simulink library "aoc"  (Simulink 8.1)
settings: Solver=ode45  StartTime=0.0  StopTime=10.0  RelTol=1e-3
settings Model: Creator=xsellart  LastModifiedBy=AT015555

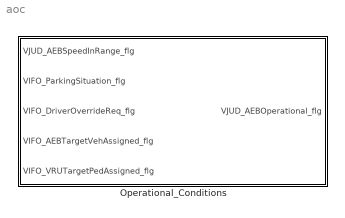
== system aoc ==
  Operational_Conditions : Subsystem

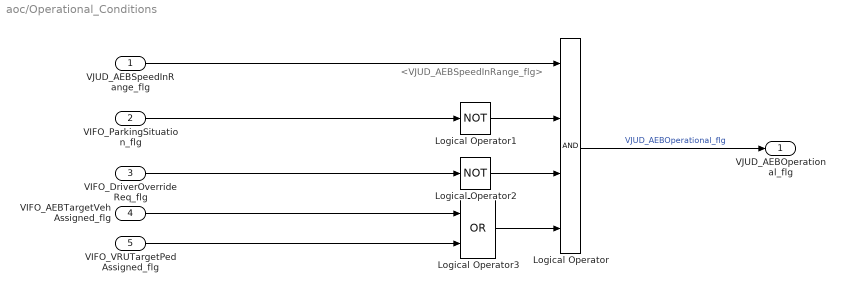
== system aoc/Operational_Conditions ==
  note: <VJUD_AEBSpeedInRange_flg>
  VJUD_AEBSpeedInRange_flg : Inport
  VIFO_ParkingSituation_flg : Inport  Port=2
  VIFO_DriverOverrideReq_flg : Inport  Port=3
  VIFO_AEBTargetVehAssigned_flg : Inport  Port=4
  VIFO_VRUTargetPedAssigned_flg : Inport  Port=5
  Logical Operator : Logic  Inputs=4  AllPortsSameDT=off  OutDataTypeStr=boolean
  Logical Operator1 : Logic  Operator=NOT  AllPortsSameDT=off  OutDataTypeStr=boolean
  Logical Operator2 : Logic  Operator=NOT  AllPortsSameDT=off  OutDataTypeStr=boolean
  Logical Operator3 : Logic  Operator=OR  AllPortsSameDT=off  OutDataTypeStr=boolean
  VJUD_AEBOperational_flg : Outport
  wires:
  VJUD_AEBSpeedInRange_flg/1 -> Logical Operator/1
  Logical Operator/1 -> VJUD_AEBOperational_flg/1  "VJUD_AEBOperational_flg"
  Logical Operator2/1 -> Logical Operator/3
  Logical Operator1/1 -> Logical Operator/2
  VIFO_DriverOverrideReq_flg/1 -> Logical Operator2/1
  VIFO_ParkingSituation_flg/1 -> Logical Operator1/1
  VIFO_AEBTargetVehAssigned_flg/1 -> Logical Operator3/1
  VIFO_VRUTargetPedAssigned_flg/1 -> Logical Operator3/2
  Logical Operator3/1 -> Logical Operator/4
